simulink model "eqns_motion_mdl"  (R2018b)
settings: Solver=VariableStepAuto  StartTime=0.0  StopTime=200  FixedStep=0.001  RelTol=1e-4
values from neighbouring files (symbols this model uses):
  air_data = load('air_data.csv')    [Saturn_V_Comp2.m]    (also in eqns_motion_script.m)
  burn_time = 153.82    [Saturn_V_Comp2.m]    (also in eqns_motion_script.m = 39.2157)
  cp = 0.217    [Saturn_V_Comp2.m]    (also in draw_vehicle.m = -aero_statdyn.xcp(alpha, 1)*aero_statdyn.cbar + vehicle.xcg; eqns_motion_script.m)
  d = 16    [Saturn_V_Comp2.m]    (also in eqns_motion_script.m)
  De = 12.2*12    (= 146.4)    [Saturn_V_Comp2.m]    (also in eqns_motion_script.m = 8.4932)
  h0 = 10    [Saturn_V_Comp2.m]    (also in eqns_motion_script.m = 4595)
  I = [360, 0, 0; 0, 4880, 0; 0, 0, 4880]./973.065    [Saturn_V_Comp2.m]    (also in eqns_motion_script.m)
  k_he = 0.0867    [Saturn_V_Comp2.m]    (also in eqns_motion_script.m)
  kc = 1    [Saturn_V_Comp2.m]    (also in eqns_motion_script.m)
  lat = 32.9861    [Saturn_V_Comp2.m]    (also in eqns_motion_script.m)
  len = 27    [Saturn_V_Comp2.m]    (also in eqns_motion_script.m)
  lon = -106.9717    [Saturn_V_Comp2.m]    (also in eqns_motion_script.m)
  lr = 75    [Saturn_V_Comp2.m]    (also in eqns_motion_script.m)
  m_dry = 1.7664E6    (= 1766400)    [Saturn_V_Comp2.m]    (also in eqns_motion_script.m = 488.705562)
  m_wet = 6132585    [Saturn_V_Comp2.m]    (also in eqns_motion_script.m = 1404)
  material_density = 168.55    [Saturn_V_Comp2.m]    (also in eqns_motion_script.m)
  mu = 0.42    [Saturn_V_Comp2.m]    (also in eqns_motion_script.m)
  Pe = 13.3069    [Saturn_V_Comp2.m]    (also in eqns_motion_script.m = 10)
  phi0 = 0    [Saturn_V_Comp2.m]    (also in eqns_motion_script.m)
  psi0 = 0    [Saturn_V_Comp2.m]    (also in eqns_motion_script.m)
  tc = 0    [Saturn_V_Comp2.m]    (also in eqns_motion_script.m)
  theta0 = 0    [Saturn_V_Comp2.m]    (also in eqns_motion_script.m)
  u0 = 0.1    [Saturn_V_Comp2.m]    (also in eqns_motion_script.m)
  v0 = 0.0    (= 0)    [Saturn_V_Comp2.m]    (also in eqns_motion_script.m)
  w0 = 0    [Saturn_V_Comp2.m]    (also in eqns_motion_script.m)
  x = [0 10 15 20 40 60 80 100 120 140 150]    [Saturn_V_Comp2.m]    (also in draw_vehicle.m = linspace(0, vehicle.L_nc, 10)'; eqns_motion_script.m = 50.61)
undefined symbols (not defined in the file or in its folder): day, Dt, Earth, mdot, Pc, Receive, sec, Send, Thrust, WGS84
libraries: aerolibconvert2 x8, simulink_extras x5, vrlib x3, simulink x3, aerolibfltsims x2, aerolibasang x2, aerolibatmos2 x1, aerolibutil x1, aerolibtransform2 x1, aerolibadyn x1, sharedtransform x1, sharedutil x1
settings Model: Creator=Arthur de Waleffe  LastModifiedBy=bartk

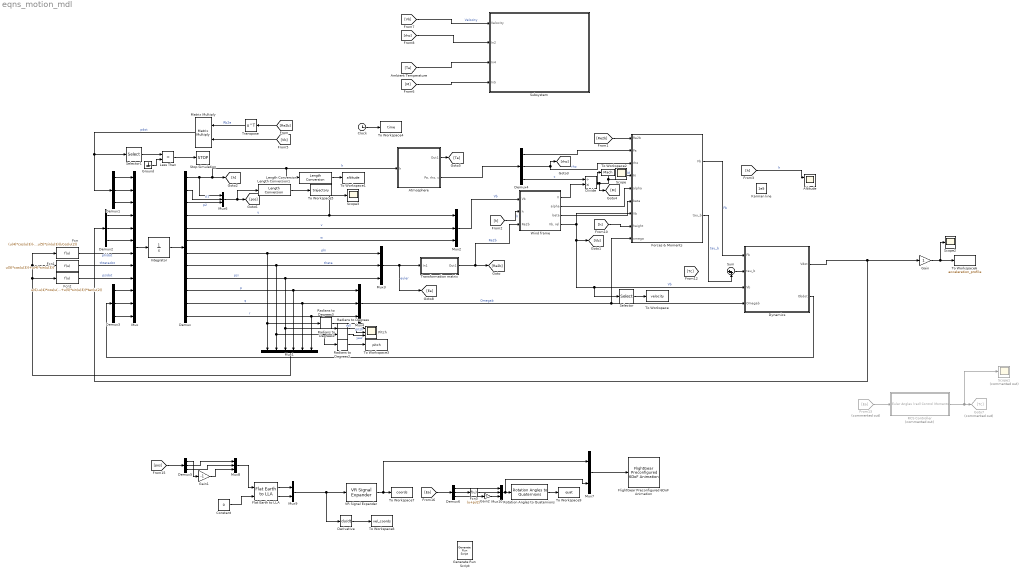
== system eqns_motion_mdl ==
  Altitude : Scope  NumInputPorts=2
  Atmosphere : Subsystem
  Clock : Clock
  Constant : Constant  Value=0
  Demux : Demux  Outputs=12
  Demux{1..6} (6 alike) : Demux  Outputs=3
  Derivative : Derivative
  Divide : Product  Inputs=/*
  Dynamics : Subsystem
  Fcn : Fcn  Expr=(u(4)*cos(u(3))-u(5)*sin(u(3)))/cos(u(2))
  Fcn1 : Fcn  Expr=u(5)*cos(u(3))+u(4)*sin(u(3))
  Fcn2 : Fcn  Expr=u(6)-u(4)*cos(u(3))*tan(u(2))+u(5)*sin(u(3))*tan(u(2))
  Fcn3 : Fcn  Expr=(u+pi/2)
  Flat Earth to LLA : aerolibtransform2/Flat Earth to LLA  units=Metric (MKS)  ptype=Earth (WGS84)  F=1/298.257223563  R=6378137  LL0=[lat lon]  psi=0
  FlightGear Preconfigured 6DoF Animation : aerolibfltsims/FlightGear Preconfigured 6DoF Animation  xFlightGearVersion=v2018.1  DestinationIpAddress=127.0.0.1  DestinationPort=5502  SampleTime=1/30  packetVersion=24
      settings: SourceProductName=Aerospace Blockset
  Forces & Moments : Subsystem
  From13 : From  Commented=on  GotoTag=Ea
  Gain : Gain
  Gain1 : Gain  Gain=-1
  Gain2 : Gain  Gain=-1
  Generate Run Script : aerolibfltsims/Generate Run Script  Architecture=Win64  dataFlow=Send-Receive  GeometryModelName=c172p  AirportId=KSFO  RunwayId=10L  InitialAltitude=h0  InitialHeading=0  OffsetDistance=0  OffsetAzimuth=0  InstallScenery=on  DisableShaders=off  OriginAddress=127.0.0.1  DestinationPort=5502  OriginPort=5505  LocalAddress=127.0.0.1  OutputFileName=runfg.bat  FlightGearBaseDirectory=C:\Program Files\FlightGear 2018.3.4
  Goto7 : Goto  Commented=on  GotoTag=Tc
  Ground : Ground
  Integrator : Integrator  InitialCondition=[h0*0.3048;0;0;u0*0.3048;v0*0.3048;w0*0.3048;phi0;theta0;psi0;0;0;0]
  Karman line : Constant  Value=1e5
  Length Conversion : aerolibconvert2/Length Conversion  IU=m  OU=ft
  Length Conversion1 : aerolibconvert2/Length Conversion  IU=m  OU=ft
  Less Than : RelationalOperator  Operator=<  OutDataTypeStr=boolean  RndMeth=Simplest
  Matrix Multiply : Product  Multiplication=Matrix(*)
  Mux : Mux  Inputs=12
  Mux1 : Mux  Inputs=6
  Mux{2..4,6,8,10} (6 alike) : Mux  Inputs=3
  Mux7 : Mux  Inputs=2
  Mux9 : Mux  Inputs=2
  Pitch : Scope  NumInputPorts=3
  RCS Controller : Subsystem  Commented=on
  Radians to Degrees{,1..3} (4 alike) : simulink_extras/Transformations/Radians to Degrees
  Rotation Angles to Quaternions : sharedtransform/Rotation Angles to Quaternions  rotationOrder=ZYX  aMode=aMode
      settings: SourceProductName=Aerospace Blockset  SourceProductBaseCode=AE
  Scope : Scope
  Scope1 : Scope  Commented=on
  Scope2 : Scope
  Scope3 : Scope
  Selector : Selector  InputPortWidth=3  IndexOptions=Index vector (dialog)  Indices=[1]  OutputSizes=1
  Selector1 : Selector  InputPortWidth=3  IndexOptions=Index vector (dialog)  Indices=[1]  OutputSizes=1
  Stop Simulation : Stop
  Subsystem : Subsystem
  Sum : Sum  Inputs=|++
  To Workspace : ToWorkspace  VariableName=velocity  SaveFormat=Timeseries  SampleTime=-1
  To Workspace1 : ToWorkspace  VariableName=altitude  SaveFormat=Timeseries  SampleTime=-1
  To Workspace2 : ToWorkspace  VariableName=Mach  SaveFormat=Timeseries  SampleTime=-1
  To Workspace3 : ToWorkspace  VariableName=pitch  SaveFormat=Timeseries  SampleTime=-1
  To Workspace4 : ToWorkspace  VariableName=time  SampleTime=-1
  To Workspace5 : ToWorkspace  VariableName=trajectory  SaveFormat=Timeseries  SampleTime=-1
  To Workspace6 : ToWorkspace  VariableName=acceleration_profile  SampleTime=-1
  To Workspace7 : ToWorkspace  VariableName=coords  SaveFormat=Structure With Time  SampleTime=-1
  To Workspace8 : ToWorkspace  VariableName=vel_coords  SaveFormat=Structure With Time  SampleTime=-1
  To Workspace9 : ToWorkspace  VariableName=quat  SaveFormat=Structure With Time  SampleTime=-1
  Transformation matrix : Subsystem
  Transpose : Math  Operator=transpose  SaturateOnIntegerOverflow=on
  VR Signal Expander : vrlib/VR Signal Expander  outwidth=3  outidx=[2 1 3]
      settings: SourceProductName=Simulink 3D Animation  SourceProductBaseCode=VR
  "Wind frame " : Subsystem
  wires:
  Integrator/1 -> Demux/1
  Mux/1 -> Integrator/1
  Demux/4 -> Scope3/1, Mux2/1  "u"
  Demux/5 -> Mux2/2  "v"
  Demux/6 -> Mux2/3  "w"
  Demux/7 -> Mux3/1, Mux1/1, Radians to Degrees3/1  "phi"
  Demux/8 -> Mux3/2, Radians to Degrees2/1, Radians to Degrees1/1, Mux1/2  "theta"
  Demux/9 -> Mux3/3, Mux1/3, Radians to Degrees/1  "psi"
  Demux/10 -> Mux4/1, Mux1/4  "p"
  Demux/12 -> Mux4/3, Mux1/6  "r"
  Demux/11 -> Mux4/2, Mux1/5  "q"
  Fcn/1 -> Mux/7  "phidot"
  Fcn1/1 -> Mux/8  "thtetadot"
  Fcn2/1 -> Mux/9  "psidot"
  Mux1/1 -> Fcn2/1, Fcn/1, Fcn1/1
  Mux3/1 -> [Ea], Transformation matrix/1(In1)  "euler"
  Transpose/1 -> Matrix Multiply/1  "Rb2e"
  Matrix Multiply/1 -> Selector1/1, Demux1/1  "pdot"
  Demux1/2 -> Mux/2
  Demux1/1 -> Mux/1
  Demux1/3 -> Mux/3
  Demux2/1 -> Mux/4
  Demux2/2 -> Mux/5
  Demux2/3 -> Mux/6
  Demux4/2 -> [rho], Forces & Moments/3(rho)  "rho"
  Demux3/1 -> Mux/10
  Demux3/2 -> Mux/11
  Demux3/3 -> Mux/12
  Demux4/3 -> Divide/1  "c"
  Divide/1 -> To Workspace2/1, [M], Scope/1, Forces & Moments/4(M)  "M"
  "Wind frame "/1(V) -> Divide/2
  "Wind frame "/2(alpha) -> Forces & Moments/5(alpha)
  "Wind frame "/3(beta) -> Forces & Moments/6(beta)
  Demux/2 -> Mux6/2  "p1"
  Demux/3 -> Mux6/3  "p2"
  Forces & Moments/1(Fb) -> Dynamics/1(Fb)  "Fb"
  Mux4/1 -> Forces & Moments/9(omega), Dynamics/4(Omegab)  "Omegab"
  Transformation matrix/1(Out1) -> "Wind frame "/3(Re2b), [Re2b]  "Re2b"
  [Re2b] -> Transpose/1
  [Re2b] -> Forces & Moments/1(Re2b)
  [Vb] -> Matrix Multiply/2
  [h] -> Altitude/1  "h"
  "Wind frame "/4("Vb, rel") -> [Vb], Selector/1, Dynamics/3(Vb), Forces & Moments/7(Vb)  "Vb"
  Mux2/1 -> "Wind frame "/1(Vb)  "Vb"
  Demux4/1 -> Forces & Moments/2(Pa)
  Atmosphere/2("Pa, rho, c") -> Demux4/1
  Demux/1 -> Mux6/1, Length Conversion/1, Atmosphere/1(h), [h]  "h"
  [h] -> "Wind frame "/2(h)  "h"
  [Ta] -> Subsystem/3(In4)
  [Vb] -> Subsystem/1(Velocity)  "Velocity"
  [M] -> Subsystem/4(In5)
  [rho] -> Subsystem/2(In2)
  Atmosphere/1(Out1) -> [Ta]
  [h] -> Forces & Moments/8(height)
  Mux6/1 -> Length Conversion1/1, [pos]
  Radians to Degrees/1 -> Pitch/2  "pitch"
  Radians to Degrees1/1 -> Pitch/3  "yaw"
  Radians to Degrees2/1 -> To Workspace3/1
  Clock/1 -> To Workspace4/1
  From13/1 -> RCS Controller/1(Euler Angles (rad))
  Dynamics/2(Obdot) -> Demux3/1
  RCS Controller/1(Control Moments) -> Scope1/1, Goto7/1
  Sum/1 -> Dynamics/2(tau_b)
  Selector/1 -> To Workspace/1
  Dynamics/1(Vdot) -> Demux2/1, Gain/1
  Gain/1 -> Scope2/1, To Workspace6/1
  Constant/1 -> Flat Earth to LLA/2
  [pos] -> Demux5/1
  Demux5/2 -> Mux8/1
  Demux5/3 -> Mux8/2
  Demux5/1 -> Gain1/1
  Gain1/1 -> Mux8/3
  Mux8/1 -> Flat Earth to LLA/1
  Flat Earth to LLA/1 -> Mux9/1
  Flat Earth to LLA/2 -> Mux9/2
  Mux9/1 -> Derivative/1, VR Signal Expander/1
  Derivative/1 -> To Workspace8/1
  [Ea] -> Demux6/1
  Demux6/1 -> Mux10/1
  Mux10/1 -> Mux7/2, Rotation Angles to Quaternions/1
  Demux6/2 -> Fcn3/1
  Demux6/3 -> Gain2/1
  Fcn3/1 -> Mux10/2
  Gain2/1 -> Mux10/3
  Ground/1 -> Less Than/2
  Less Than/1 -> Stop Simulation/1
  Rotation Angles to Quaternions/1 -> To Workspace9/1
  Radians to Degrees3/1 -> Pitch/1  "roll"
  VR Signal Expander/1 -> Mux7/1, To Workspace7/1
  Mux7/1 -> FlightGear Preconfigured 6DoF Animation/1
  Forces & Moments/2(tau_b) -> Sum/2  "tau_b"
  Length Conversion/1 -> To Workspace1/1
  Length Conversion1/1 -> To Workspace5/1
  Selector1/1 -> Less Than/1

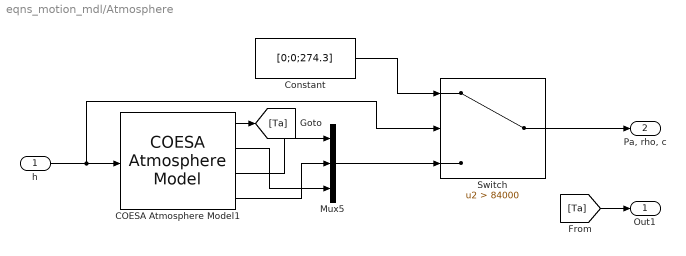
== system eqns_motion_mdl/Atmosphere ==
  h : Inport
  COESA Atmosphere Model1 : aerolibatmos2/COESA Atmosphere Model  units=Metric (MKS)  spec=1976 COESA-extended U.S. Standard Atmosphere  model=Profile  profile_var=High temperature  profile_percent=1%  profile_alt=5 km (16404 ft)  envelope_var=High temperature  envelope_percent=1%  action=Warning
  Constant : Constant  Value=[0;0;274.3]
  Mux5 : Mux  Inputs=3
  Switch : Switch  Criteria=u2 > Threshold  Threshold=84000
  Out1 : Outport
  "Pa, rho, c" : Outport  Port=2
  wires:
  Switch/1 -> "Pa, rho, c"/1
  COESA Atmosphere Model1/3 -> Mux5/1
  Constant/1 -> Switch/1
  Mux5/1 -> Switch/3
  COESA Atmosphere Model1/1 -> [Ta]
  COESA Atmosphere Model1/4 -> Mux5/2
  COESA Atmosphere Model1/2 -> Mux5/3
  h/1 -> COESA Atmosphere Model1/1, Switch/2
  [Ta] -> Out1/1

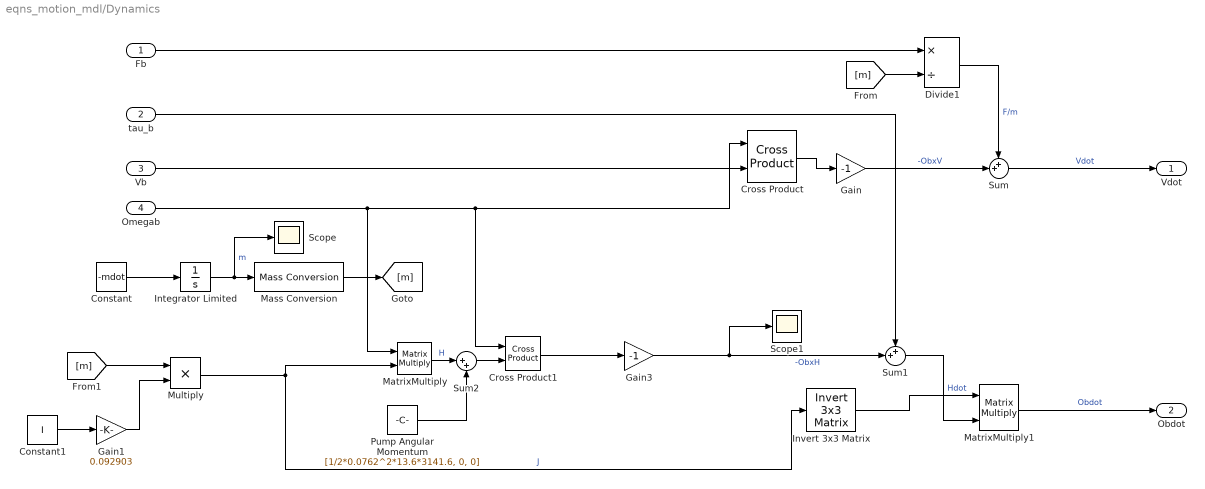
== system eqns_motion_mdl/Dynamics ==
  Fb : Inport
  tau_b : Inport  Port=2
  Vb : Inport  Port=3
  Omegab : Inport  Port=4
  Constant : Constant  Value=-mdot
  Constant1 : Constant  Value=I
  Cross Product : vrlib/Utilities/Cross Product
      settings: SourceProductBaseCode=VR
  Cross Product1 : vrlib/Utilities/Cross Product
      settings: SourceProductBaseCode=VR
  Divide1 : Product  Inputs=*/
  Gain : Gain  Gain=-1
  Gain1 : Gain  Gain=0.092903
  Gain3 : Gain  Gain=-1
  Integrator Limited : Integrator  InitialCondition=m_wet  LimitOutput=on  UpperSaturationLimit=m_wet  LowerSaturationLimit=m_dry
  Invert 3x3 Matrix : aerolibutil/Invert  3x3 Matrix
  Mass Conversion : aerolibconvert2/Mass Conversion  IU=lbm  OU=kg
      settings: SourceProductName=Aerospace Blockset  SourceProductBaseCode=AE
  MatrixMultiply : Product  Multiplication=Matrix(*)
  MatrixMultiply1 : Product  Multiplication=Matrix(*)
  Multiply : Product
  Pump Angular Momentum : Constant  Value=[1/2*0.0762^2*13.6*3141.6, 0, 0]
  Scope : Scope
  Scope1 : Scope
  Sum : Sum  Inputs=++|
  Sum1 : Sum  Inputs=++|
  Sum2 : Sum  Inputs=|++
  Vdot : Outport
  Obdot : Outport  Port=2
  wires:
  Multiply/1 -> MatrixMultiply/2, Invert 3x3 Matrix/1  "J"
  MatrixMultiply1/1 -> Obdot/1  "Obdot"
  Cross Product/1 -> Gain/1
  Sum1/1 -> MatrixMultiply1/2  "Hdot"
  Integrator Limited/1 -> Scope/1, Mass Conversion/1  "m"
  Gain3/1 -> Scope1/1, Sum1/2  "-ObxH"
  Cross Product1/1 -> Gain3/1
  Omegab/1 -> Cross Product/1, Cross Product1/1, MatrixMultiply/1
  Gain/1 -> Sum/2  "-ObxV"
  Invert 3x3 Matrix/1 -> MatrixMultiply1/1
  Sum/1 -> Vdot/1  "Vdot"
  Divide1/1 -> Sum/1  "F/m"
  Vb/1 -> Cross Product/2
  Fb/1 -> Divide1/1
  tau_b/1 -> Sum1/1
  [m] -> Divide1/2
  [m] -> Multiply/1
  Constant/1 -> Integrator Limited/1
  MatrixMultiply/1 -> Sum2/1  "H"
  Sum2/1 -> Cross Product1/2
  Pump Angular Momentum/1 -> Sum2/2
  Mass Conversion/1 -> [m]
  Constant1/1 -> Gain1/1
  Gain1/1 -> Multiply/2

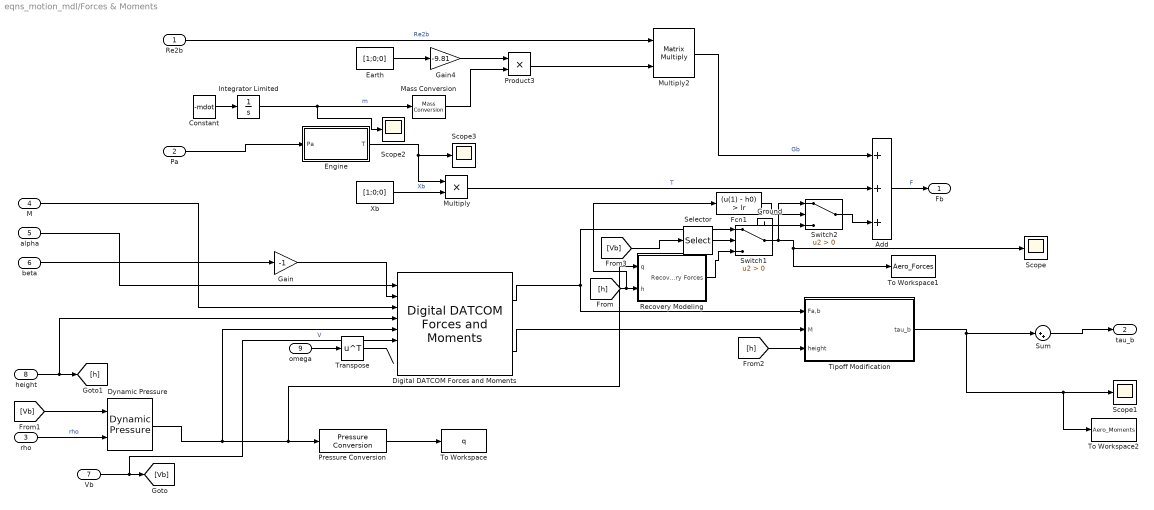
== system eqns_motion_mdl/Forces & Moments ==
  Re2b : Inport
  Pa : Inport  Port=2
  rho : Inport  Port=3
  M : Inport  Port=4
  alpha : Inport  Port=5
  beta : Inport  Port=6
  Vb : Inport  Port=7
  height : Inport  Port=8
  omega : Inport  Port=9
  Add : Sum  Inputs=+++
  Constant : Constant  Value=-mdot
  Digital DATCOM Forces and Moments : aerolibadyn/Digital DATCOM Forces and Moments  units=Metric (MKS)  dcase=aero_statdyn  fmode=Body  buildno=0  imethod=Linear  emethod=Linear  rmethod=Linear Extrapolation  action=None
      settings: SourceProductName=Aerospace Blockset  SourceProductBaseCode=AE
  Dynamic Pressure : aerolibasang/Dynamic Pressure
  Earth : Constant  Value=[1;0;0]
  Engine : Subsystem
  Fcn1 : Fcn  Expr=(u(1) - h0) > lr
  Gain : Gain  Gain=-1
  Gain4 : Gain  Gain=-9.81
  Ground : Ground
  Integrator Limited : Integrator  InitialCondition=m_wet  LimitOutput=on  UpperSaturationLimit=m_wet  LowerSaturationLimit=m_dry
  Mass Conversion : aerolibconvert2/Mass Conversion  IU=lbm  OU=kg
      settings: SourceProductName=Aerospace Blockset  SourceProductBaseCode=AE
  Multiply : Product
  Multiply2 : Product  Multiplication=Matrix(*)
  Pressure Conversion : aerolibconvert2/Pressure Conversion  IU=Pa  OU=psf
      settings: SourceProductName=Aerospace Blockset  SourceProductBaseCode=AE
  Product3 : Product
  Recovery Modeling : Subsystem
  Scope{,1..3} (4 alike) : Scope
  Selector : Selector  InputPortWidth=3  IndexOptions=Index vector (dialog)  Indices=[1]  OutputSizes=1
  Sum : Sum  Inputs=|++
  Switch1 : Switch  Criteria=u2 > Threshold
  Switch2 : Switch  Criteria=u2 > Threshold
  Tipoff Modification : Subsystem
  To Workspace : ToWorkspace  VariableName=q  SaveFormat=Timeseries  SampleTime=-1
  To Workspace1 : ToWorkspace  VariableName=Aero_Forces  SaveFormat=Timeseries  SampleTime=-1
  To Workspace2 : ToWorkspace  VariableName=Aero_Moments  SaveFormat=Timeseries  SampleTime=-1
  Transpose : Math  Operator=transpose  SaturateOnIntegerOverflow=on
  Xb : Constant  Value=[1;0;0]
  Fb : Outport
  tau_b : Outport  Port=2
  wires:
  Multiply2/1 -> Add/1  "Gb"
  Re2b/1 -> Multiply2/1  "Re2b"
  Earth/1 -> Gain4/1
  Add/1 -> Fb/1  "F"
  Gain4/1 -> Product3/1
  Integrator Limited/1 -> Mass Conversion/1, Scope2/1  "m"
  Product3/1 -> Multiply2/2
  Xb/1 -> Multiply/2  "Xb"
  Multiply/1 -> Add/2  "T"
  rho/1 -> Dynamic Pressure/2  "rho"
  [Vb] -> Dynamic Pressure/1
  Pa/1 -> Engine/1(Pa)
  Engine/1(T) -> Scope3/1, Multiply/1
  [h] -> Tipoff Modification/3(height)
  height/1 -> Digital DATCOM Forces and Moments/4, [h]
  Vb/1 -> Digital DATCOM Forces and Moments/6, [Vb]  "V"
  Dynamic Pressure/1 -> Digital DATCOM Forces and Moments/5, Recovery Modeling/1(q), Pressure Conversion/1
  M/1 -> Digital DATCOM Forces and Moments/3
  alpha/1 -> Digital DATCOM Forces and Moments/1
  beta/1 -> Gain/1
  Gain/1 -> Digital DATCOM Forces and Moments/2
  omega/1 -> Transpose/1
  Digital DATCOM Forces and Moments/2 -> Tipoff Modification/2(M)
  Digital DATCOM Forces and Moments/1 -> Switch1/1, Tipoff Modification/1(Fa,b)
  Transpose/1 -> ?
  Tipoff Modification/1(tau_b) -> Sum/1, Scope1/1, To Workspace2/1
  Switch1/1 -> Switch2/1, To Workspace1/1, Scope/1
  Recovery Modeling/1(Recovery Forces) -> Switch1/3
  [h] -> Fcn1/1, Recovery Modeling/2(h)
  [Vb] -> Selector/1
  Selector/1 -> Switch1/2
  Pressure Conversion/1 -> To Workspace/1
  Fcn1/1 -> Switch2/2
  Ground/1 -> Switch2/3
  Constant/1 -> Integrator Limited/1
  Mass Conversion/1 -> Product3/2
  Switch2/1 -> Add/3
  Sum/1 -> tau_b/1

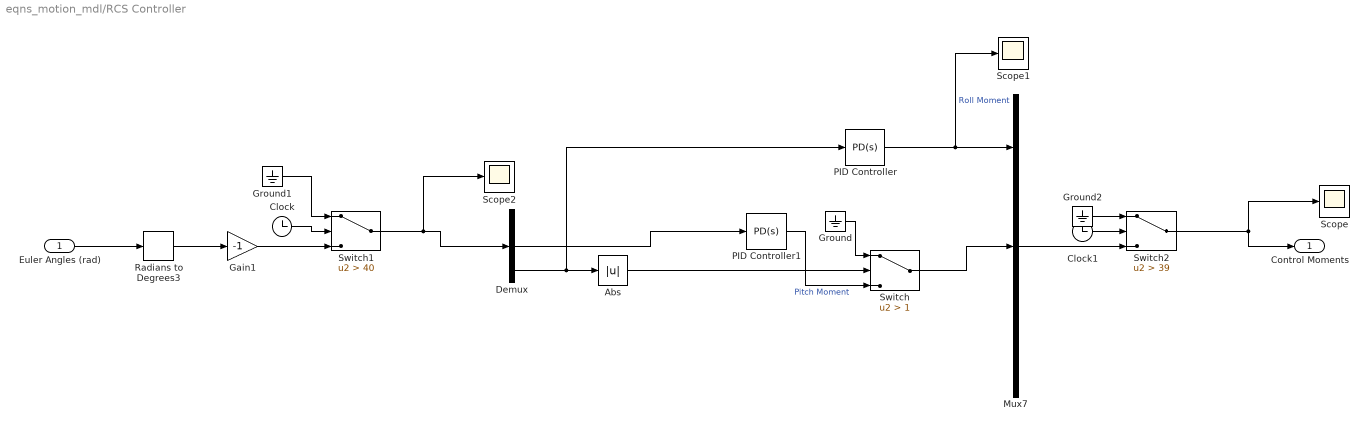
== system eqns_motion_mdl/RCS Controller ==
  Euler Angles (rad) : Inport
  Abs : Abs
  Clock : Clock
  Clock1 : Clock
  Demux : Demux  Outputs=3
  Gain1 : Gain  Gain=-1
  Ground : Ground
  Ground1 : Ground
  Ground2 : Ground
  Mux7 : Mux  Inputs=3
  PID Controller : simulink/Continuous/PID Controller  Controller=PD  Form=Parallel  TimeDomain=Continuous-time  SampleTime=-1  IntegratorMethod=Forward Euler  FilterMethod=Forward Euler  ControllerParametersSource=internal  P=2  I=1  D=2  UseFilter=on  N=100  TunerSelectOption=Transfer Function Based (PID Tuner App)  InitialConditionSource=internal  InitialConditionForIntegrator=0  InitialConditionForFilter=0  DifferentiatorICPrevScaledInput=0  ExternalReset=none  TrackingMode=off  Kt=1  LimitOutput=off  UpperSaturationLimit=inf  LowerSaturationLimit=-inf  LinearizeAsGain=on  AntiWindupMode=none  Kb=1  POutMin=[]  POutMax=[]  IOutMin=[]  IOutMax=[]  DOutMin=[]  DOutMax=[]  NOutMin=[]  NOutMax=[]  SumOutMin=[]  SumOutMax=[]  SaturationOutMin=[]  SaturationOutMax=[]  PParamMin=[]  PParamMax=[]  IParamMin=[]  IParamMax=[]  DParamMin=[]  DParamMax=[]  NParamMin=[]  NParamMax=[]  KbParamMin=[]  KbParamMax=[]  KtParamMin=[]  KtParamMax=[]  KbOutMin=[]  KbOutMax=[]  KtOutMin=[]  KtOutMax=[]  IntegratorOutMin=[]  IntegratorOutMax=[]  FilterOutMin=[]  FilterOutMax=[]  SumI1OutMin=[]  SumI1OutMax=[]  SumI2OutMin=[]  SumI2OutMax=[]  SumI3OutMin=[]  SumI3OutMax=[]  SumI4OutMin=[]  SumI4OutMax=[]  SumDOutMin=[]  SumDOutMax=[]  DifferentiatorOutMin=[]  DifferentiatorOutMax=[]  FilterDiffOutCoefMin=[]  FilterDiffOutCoefMax=[]  ReciprocalOutMin=[]  ReciprocalOutMax=[]  SumDenOutMin=[]  SumDenOutMax=[]  SumNumOutMin=[]  SumNumOutMax=[]  DivideOutMin=[]  DivideOutMax=[]  IntegratorContinuousStateAttributes=''  IntegratorStateMustResolveToSignalObject=off  IntegratorRTWStateStorageClass=Auto  FilterContinuousStateAttributes=''  FilterStateMustResolveToSignalObject=off  FilterRTWStateStorageClass=Auto  ParallelPVariant=InternalParameters  IdealPVariant=Disabled  IVariant=Disabled  DVariant=InternalParameters  IntegratorVariant=Disabled  SatVariant=Disabled  AWVariant=Disabled  PCopyVariant=Disabled  TRVariant=Disabled  FdbkBlocksVariant=Forward  IdealPFdbkVariant=Disabled  SatFdbkVariant=Disabled  DerivativeFilterVariant=ContFilter  NVariant=InternalParameters  NCopyVariant=Disabled  FilterICVariant=InternalICsFilter  IntegratorICVariant=Disabled  ExternalResetVariant=Disabled  TRSumVariant=Passthrough  SumFdbkVariant=Disabled  SumVariant=Sum_PD
  PID Controller1 : simulink/Continuous/PID Controller  Controller=PD  Form=Parallel  TimeDomain=Continuous-time  SampleTime=-1  IntegratorMethod=Forward Euler  FilterMethod=Forward Euler  ControllerParametersSource=internal  P=1281.40350850482  I=1  D=624.70270979077  UseFilter=on  N=100  TunerSelectOption=Transfer Function Based (PID Tuner App)  InitialConditionSource=internal  InitialConditionForIntegrator=0  InitialConditionForFilter=0  DifferentiatorICPrevScaledInput=0  ExternalReset=none  TrackingMode=off  Kt=1  LimitOutput=on  UpperSaturationLimit=1000  LowerSaturationLimit=-1000  LinearizeAsGain=on  AntiWindupMode=none  Kb=1  POutMin=[]  POutMax=[]  IOutMin=[]  IOutMax=[]  DOutMin=[]  DOutMax=[]  NOutMin=[]  NOutMax=[]  SumOutMin=[]  SumOutMax=[]  SaturationOutMin=[]  SaturationOutMax=[]  PParamMin=[]  PParamMax=[]  IParamMin=[]  IParamMax=[]  DParamMin=[]  DParamMax=[]  NParamMin=[]  NParamMax=[]  KbParamMin=[]  KbParamMax=[]  KtParamMin=[]  KtParamMax=[]  KbOutMin=[]  KbOutMax=[]  KtOutMin=[]  KtOutMax=[]  IntegratorOutMin=[]  IntegratorOutMax=[]  FilterOutMin=[]  FilterOutMax=[]  SumI1OutMin=[]  SumI1OutMax=[]  SumI2OutMin=[]  SumI2OutMax=[]  SumI3OutMin=[]  SumI3OutMax=[]  SumI4OutMin=[]  SumI4OutMax=[]  SumDOutMin=[]  SumDOutMax=[]  DifferentiatorOutMin=[]  DifferentiatorOutMax=[]  FilterDiffOutCoefMin=[]  FilterDiffOutCoefMax=[]  ReciprocalOutMin=[]  ReciprocalOutMax=[]  SumDenOutMin=[]  SumDenOutMax=[]  SumNumOutMin=[]  SumNumOutMax=[]  DivideOutMin=[]  DivideOutMax=[]  IntegratorContinuousStateAttributes=''  IntegratorStateMustResolveToSignalObject=off  IntegratorRTWStateStorageClass=Auto  FilterContinuousStateAttributes=''  FilterStateMustResolveToSignalObject=off  FilterRTWStateStorageClass=Auto  ParallelPVariant=InternalParameters  IdealPVariant=Disabled  IVariant=Disabled  DVariant=InternalParameters  IntegratorVariant=Disabled  SatVariant=Enabled  AWVariant=Disabled  PCopyVariant=Disabled  TRVariant=Disabled  FdbkBlocksVariant=Forward  IdealPFdbkVariant=Disabled  SatFdbkVariant=Disabled  DerivativeFilterVariant=ContFilter  NVariant=InternalParameters  NCopyVariant=Disabled  FilterICVariant=InternalICsFilter  IntegratorICVariant=Disabled  ExternalResetVariant=Disabled  TRSumVariant=Passthrough  SumFdbkVariant=Disabled  SumVariant=Sum_PD
  Radians to Degrees3 : simulink_extras/Transformations/Radians to Degrees
  Scope : Scope
  Scope1 : Scope
  Scope2 : Scope
  Switch : Switch  Criteria=u2 > Threshold  Threshold=1
  Switch1 : Switch  Criteria=u2 > Threshold  Threshold=40
  Switch2 : Switch  Criteria=u2 > Threshold  Threshold=39
  Control Moments : Outport
  wires:
  Radians to Degrees3/1 -> Gain1/1
  PID Controller/1 -> Scope1/1, Mux7/1  "Roll Moment"
  Euler Angles (rad)/1 -> Radians to Degrees3/1
  Demux/2 -> PID Controller1/1
  PID Controller1/1 -> Switch/3  "Pitch Moment"
  Ground/1 -> Switch/1
  Demux/3 -> PID Controller/1, Abs/1
  Abs/1 -> Switch/2
  Switch/1 -> Mux7/2
  Gain1/1 -> Switch1/3
  Switch1/1 -> Scope2/1, Demux/1
  Clock/1 -> Switch1/2
  Ground1/1 -> Switch1/1
  Mux7/1 -> Switch2/3
  Switch2/1 -> Control Moments/1, Scope/1
  Clock1/1 -> Switch2/2
  Ground2/1 -> Switch2/1

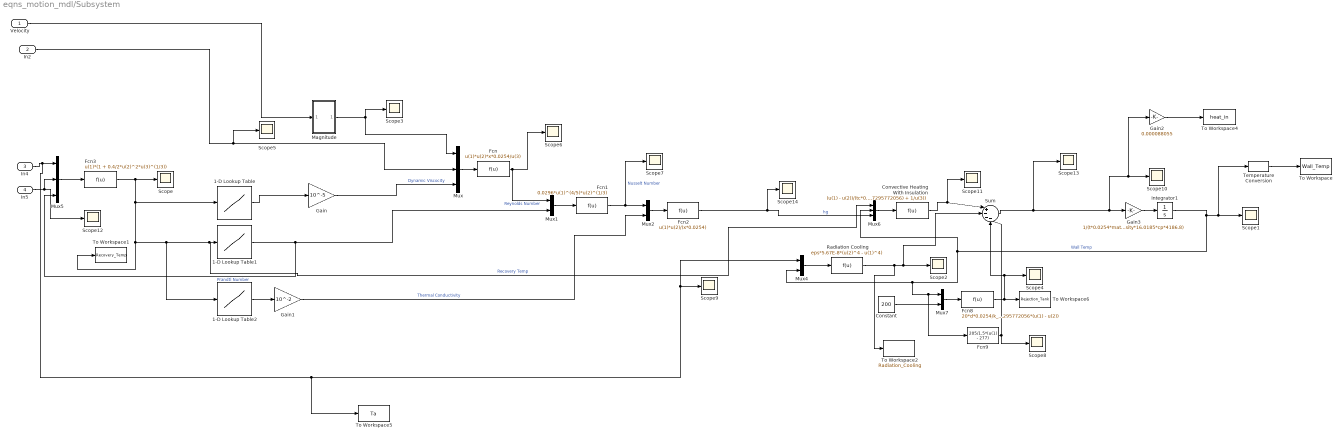
== system eqns_motion_mdl/Subsystem ==
  Velocity : Inport
  In2 : Inport  Port=2
  In4 : Inport  Port=3
  In5 : Inport  Port=4
  1-D Lookup Table : Lookup_n-D  NumberOfTableDimensions=1  BreakpointsForDimension1=air_data(:,1)  Table=air_data(:,5)  InternalRulePriority=Speed  RndMeth=Simplest  InputSameDT=on
  1-D Lookup Table1 : Lookup_n-D  NumberOfTableDimensions=1  BreakpointsForDimension1=air_data(:,1)  Table=air_data(:,7)  InternalRulePriority=Speed  RndMeth=Simplest  InputSameDT=on
  1-D Lookup Table2 : Lookup_n-D  NumberOfTableDimensions=1  BreakpointsForDimension1=air_data(:,1)  Table=air_data(:,6)  InternalRulePriority=Speed  RndMeth=Simplest  InputSameDT=on
  Constant : Constant  Value=200
  Convective Heating With Insulation : Fcn  Expr=(u(1) - u(2))/(tc*0.0254/(kc*1.7295772056) + 1/u(3))
  Fcn : Fcn  Expr=u(1)*u(2)*x*0.0254/u(3)
  Fcn1 : Fcn  Expr=0.0296*u(1)^(4/5)*u(2)^(1/3)
  Fcn2 : Fcn  Expr=u(1)*u(2)/(x*0.0254)
  Fcn3 : Fcn  Expr=u(1)*(1 + 0.4/2*u(2)^2*u(3)^(1/3))
  Fcn8 : Fcn  Expr=20*d*0.0254/k_he/1.7295772056*(u(1) - u(2))
  Fcn9 : Fcn  Expr=205/1.5*(u(1) - 277)
  Gain : Gain  Gain=10^-5
  Gain1 : Gain  Gain=10^-2
  Gain2 : Gain  Gain=0.000088055
  Gain3 : Gain  Gain=1/(t*0.0254*material_density*16.0185*cp*4186.8)
  Integrator1 : Integrator  InitialCondition=277
  Magnitude : Subsystem
  Mux : Mux  Inputs=3
  Mux{1..2,4,7} (4 alike) : Mux  Inputs=2
  Mux5 : Mux  Inputs=3
  Mux6 : Mux  Inputs=3
  Radiation Cooling : Fcn  Expr=eps*5.67E-8*(u(2)^4 - u(1)^4)
  Scope{,1..14} (15 alike) : Scope
  Sum : Sum  Inputs=|+---
  Temperature Conversion : aerolibconvert2/Temperature Conversion  IU=K  OU=F
      settings: SourceProductName=Aerospace Blockset  SourceProductBaseCode=AE
  To Workspace : ToWorkspace  VariableName=Wall_Temp  SaveFormat=Timeseries  SampleTime=-1
  To Workspace1 : ToWorkspace  VariableName=Recovery_Temp  SaveFormat=Timeseries  SampleTime=-1
  To Workspace2 : ToWorkspace  VariableName=Radiation_Cooling  SaveFormat=Timeseries  SampleTime=-1
  To Workspace4 : ToWorkspace  VariableName=heat_in  SaveFormat=Structure With Time  SampleTime=-1
  To Workspace5 : ToWorkspace  VariableName=Ta  SaveFormat=Timeseries  SampleTime=-1
  To Workspace6 : ToWorkspace  VariableName=Rejection_Tank  SaveFormat=Timeseries  SampleTime=-1
  wires:
  Gain1/1 -> Mux2/2  "Thermal Conductivity"
  Mux5/1 -> Fcn3/1
  Fcn3/1 -> To Workspace1/1, 1-D Lookup Table2/1, Mux6/1, 1-D Lookup Table1/1, 1-D Lookup Table/1, Scope/1  "Recovery Temp"
  1-D Lookup Table1/1 -> Mux1/2, Mux5/3  "Prandtl Number"
  In2/1 -> Mux/2, Scope5/1
  1-D Lookup Table2/1 -> Gain1/1
  Gain/1 -> Mux/3  "Dynamic Viscocity"
  Integrator1/1 -> Mux6/2, Fcn9/1, Mux7/1, Mux4/2, Temperature Conversion/1, Scope1/1  "Wall Temp"
  In5/1 -> Scope12/1, Mux5/2
  Magnitude/1(Out1) -> Mux/1, Scope3/1
  1-D Lookup Table/1 -> Gain/1
  Velocity/1 -> Magnitude/1(Velocity)
  In4/1 -> To Workspace5/1, Scope9/1, Mux4/1, Mux5/1
  Mux/1 -> Fcn/1
  Fcn/1 -> Mux1/1, Scope6/1  "Reynolds Number"
  Mux1/1 -> Fcn1/1
  Fcn1/1 -> Scope7/1, Mux2/1  "Nusselt Number"
  Mux2/1 -> Fcn2/1
  Radiation Cooling/1 -> To Workspace2/1, Sum/2, Scope2/1
  Mux4/1 -> Radiation Cooling/1
  Gain3/1 -> Integrator1/1
  Convective Heating With Insulation/1 -> Scope11/1, Sum/1
  Mux6/1 -> Convective Heating With Insulation/1
  Mux7/1 -> Fcn8/1
  Fcn8/1 -> To Workspace6/1, Scope4/1, Sum/4
  Sum/1 -> Scope13/1, Gain2/1, Scope10/1, Gain3/1
  Temperature Conversion/1 -> To Workspace/1
  Gain2/1 -> To Workspace4/1
  Fcn9/1 -> Scope8/1, Sum/3
  Fcn2/1 -> Scope14/1, Mux6/3  "hg"
  Constant/1 -> Mux7/2

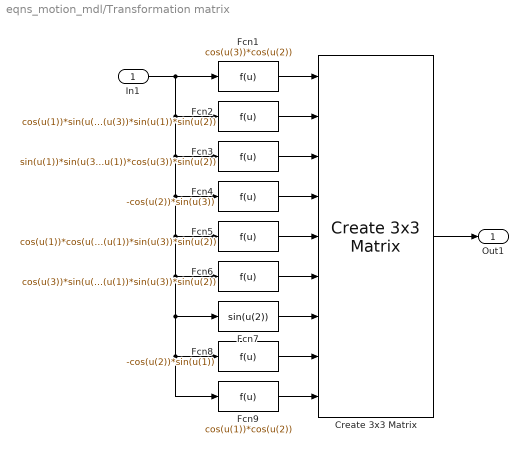
== system eqns_motion_mdl/Transformation matrix ==
  In1 : Inport
  Create 3x3 Matrix : sharedutil/Create 3x3 Matrix  aMode=aMode
  Fcn1 : Fcn  Expr=cos(u(3))*cos(u(2))
  Fcn2 : Fcn  Expr=cos(u(1))*sin(u(3)) + cos(u(3))*sin(u(1))*sin(u(2))
  Fcn3 : Fcn  Expr=sin(u(1))*sin(u(3)) - cos(u(1))*cos(u(3))*sin(u(2))
  Fcn4 : Fcn  Expr=-cos(u(2))*sin(u(3))
  Fcn5 : Fcn  Expr=cos(u(1))*cos(u(3)) - sin(u(1))*sin(u(3))*sin(u(2))
  Fcn6 : Fcn  Expr=cos(u(3))*sin(u(1)) + cos(u(1))*sin(u(3))*sin(u(2))
  Fcn7 : Fcn  Expr=sin(u(2))
  Fcn8 : Fcn  Expr=-cos(u(2))*sin(u(1))
  Fcn9 : Fcn  Expr=cos(u(1))*cos(u(2))
  Out1 : Outport
  wires:
  In1/1 -> Fcn9/1, Fcn8/1, Fcn7/1, Fcn6/1, Fcn5/1, Fcn4/1, Fcn3/1, Fcn2/1, Fcn1/1
  Fcn9/1 -> Create 3x3 Matrix/9
  Fcn8/1 -> Create 3x3 Matrix/8
  Fcn7/1 -> Create 3x3 Matrix/7
  Fcn6/1 -> Create 3x3 Matrix/6
  Fcn5/1 -> Create 3x3 Matrix/5
  Fcn4/1 -> Create 3x3 Matrix/4
  Fcn3/1 -> Create 3x3 Matrix/3
  Fcn2/1 -> Create 3x3 Matrix/2
  Fcn1/1 -> Create 3x3 Matrix/1
  Create 3x3 Matrix/1 -> Out1/1

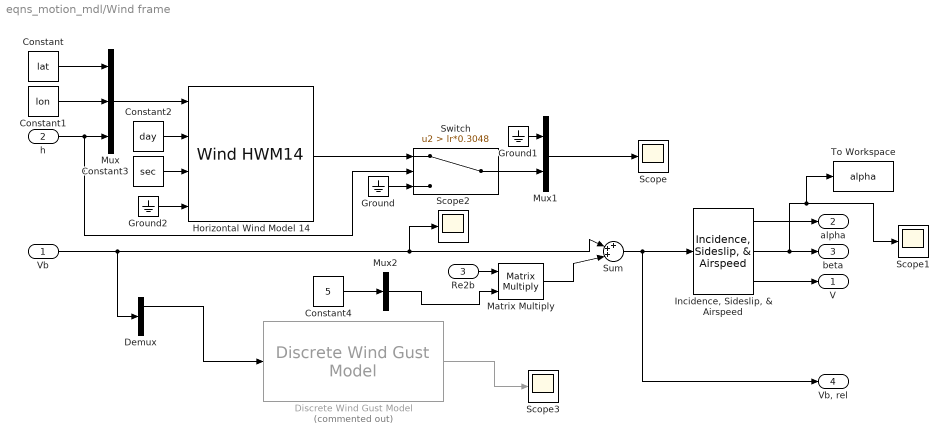
== system eqns_motion_mdl/Wind frame  ==
  Vb : Inport
  h : Inport  Port=2
  Re2b : Inport  Port=3
  Constant : Constant  Value=lat
  Constant1 : Constant  Value=lon
  Constant2 : Constant  Value=day
  Constant3 : Constant  Value=sec
  Constant4 : Constant  Value=5
  Demux : Demux  Outputs=3
  Discrete Wind Gust Model : aerolibwind2/Discrete Wind Gust Model  Commented=on  units=Metric (MKS)  Gx=off  Gy=on  Gz=off  t_0=17  d_m=[0 10 0]  v_m=[0 10 0]
      settings: SourceProductName=Aerospace Blockset
  Ground : Ground
  Ground1 : Ground
  Ground2 : Ground
  Horizontal Wind Model 14 : WindHWM14  model=Total  action=None
  "Incidence, Sideslip, & Airspeed" : aerolibasang/Incidence, Sideslip, & Airspeed
      settings: SourceProductName=Aerospace Blockset
  Matrix Multiply : Product  Multiplication=Matrix(*)
  Mux : Mux  Inputs=3
  Mux1 : Mux  Inputs=2
  Mux2 : Mux  Inputs=3
  Scope{,1..3} (4 alike) : Scope
  Sum : Sum  Inputs=+++|
  Switch : Switch  Criteria=u2 > Threshold  Threshold=lr*0.3048
  To Workspace : ToWorkspace  VariableName=alpha  SaveFormat=Timeseries  SampleTime=-1
  V : Outport
  alpha : Outport  Port=2
  beta : Outport  Port=3
  "Vb, rel" : Outport  Port=4
  wires:
  Sum/1 -> "Vb, rel"/1, "Incidence, Sideslip, & Airspeed"/1
  "Incidence, Sideslip, & Airspeed"/3 -> V/1
  "Incidence, Sideslip, & Airspeed"/1 -> alpha/1
  "Incidence, Sideslip, & Airspeed"/2 -> To Workspace/1, Scope1/1, beta/1
  h/1 -> Switch/2, Mux/3
  Mux/1 -> Horizontal Wind Model 14/1
  Constant1/1 -> Mux/2
  Constant/1 -> Mux/1
  Constant2/1 -> Horizontal Wind Model 14/2
  Constant3/1 -> Horizontal Wind Model 14/3
  Horizontal Wind Model 14/1 -> Switch/1
  Ground/1 -> Switch/3
  Switch/1 -> Mux1/2
  Ground1/1 -> Mux1/1
  Vb/1 -> Demux/1, Scope2/1, Sum/2
  Ground2/1 -> Horizontal Wind Model 14/4
  Mux1/1 -> Scope/1
  Discrete Wind Gust Model/1 -> Scope3/1
  Demux/1 -> Discrete Wind Gust Model/1
  Constant4/1 -> Mux2/2
  Re2b/1 -> Matrix Multiply/1
  Mux2/1 -> Matrix Multiply/2
  Matrix Multiply/1 -> Sum/3

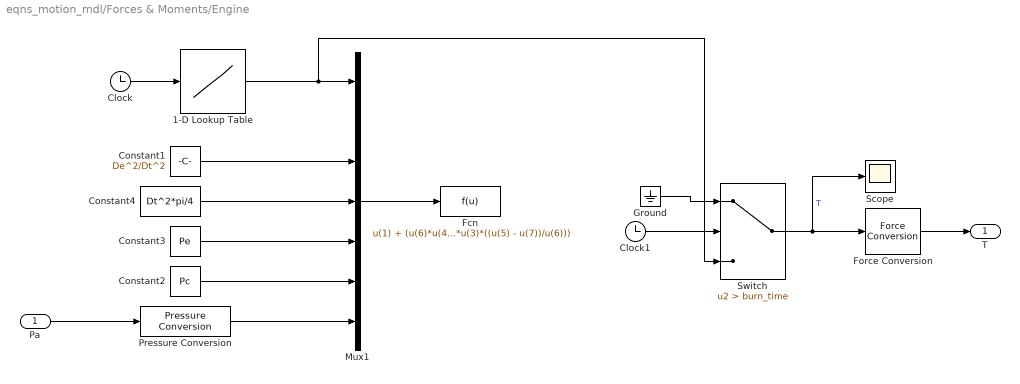
== system eqns_motion_mdl/Forces & Moments/Engine ==
  Pa : Inport
  1-D Lookup Table : Lookup_n-D  NumberOfTableDimensions=1  BreakpointsForDimension1=Thrust.time  Table=Thrust.thrust  InternalRulePriority=Speed  RndMeth=Simplest  InputSameDT=on
  Clock : Clock
  Clock1 : Clock
  Constant1 : Constant  Value=De^2/Dt^2
  Constant2 : Constant  Value=Pc
  Constant3 : Constant  Value=Pe
  Constant4 : Constant  Value=Dt^2*pi/4
  Fcn : Fcn  Expr=u(1) + (u(6)*u(4)*u(3)*((u(5) - u(7))/u(6)))
  Force Conversion : aerolibconvert2/Force Conversion  IU=lbf  OU=N
      settings: SourceProductName=Aerospace Blockset  SourceProductBaseCode=AE
  Ground : Ground
  Mux1 : Mux  Inputs=7
  Pressure Conversion : aerolibconvert2/Pressure Conversion  IU=Pa  OU=psi
      settings: SourceProductName=Aerospace Blockset  SourceProductBaseCode=AE
  Scope : Scope
  Switch : Switch  Criteria=u2 > Threshold  Threshold=burn_time
  T : Outport
  wires:
  Constant2/1 -> Mux1/6
  Constant3/1 -> Mux1/5
  Mux1/1 -> Fcn/1
  Constant1/1 -> Mux1/3
  Pa/1 -> Pressure Conversion/1
  Constant4/1 -> Mux1/4
  Switch/1 -> Force Conversion/1, Scope/1  "T"
  Force Conversion/1 -> T/1
  Pressure Conversion/1 -> Mux1/7
  Clock1/1 -> Switch/2
  Ground/1 -> Switch/1
  1-D Lookup Table/1 -> Switch/3, Mux1/1
  Clock/1 -> 1-D Lookup Table/1

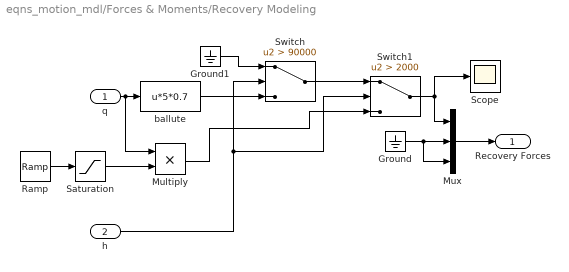
== system eqns_motion_mdl/Forces & Moments/Recovery Modeling ==
  q : Inport
  h : Inport  Port=2
  Ground : Ground
  Ground1 : Ground
  Multiply : Product
  Mux : Mux  Inputs=3
  Ramp : simulink/Sources/Ramp  slope=35.21  start=640  InitialOutput=0
  Saturation : Saturate  UpperLimit=65*0.65  LowerLimit=0
  Scope : Scope
  Switch : Switch  Criteria=u2 > Threshold  Threshold=90000
  Switch1 : Switch  Criteria=u2 > Threshold  Threshold=2000
  ballute : Fcn  Expr=u*5*0.7
  Recovery Forces : Outport
  wires:
  q/1 -> Multiply/1, ballute/1
  Mux/1 -> Recovery Forces/1
  Ground/1 -> Mux/3, Mux/2
  Ground1/1 -> Switch/1
  h/1 -> Switch1/2, Switch/2
  ballute/1 -> Switch/3
  Multiply/1 -> Switch1/3
  Switch/1 -> Switch1/1
  Switch1/1 -> Scope/1, Mux/1
  Ramp/1 -> Saturation/1
  Saturation/1 -> Multiply/2

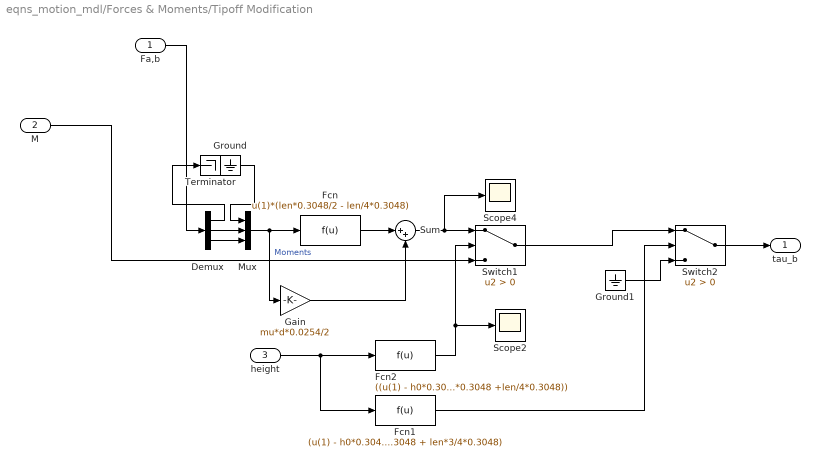
== system eqns_motion_mdl/Forces & Moments/Tipoff Modification ==
  Fa,b : Inport
  M : Inport  Port=2
  height : Inport  Port=3
  Demux : Demux  Outputs=3
  Fcn : Fcn  Expr=u(1)*(len*0.3048/2 - len/4*0.3048)
  Fcn1 : Fcn  Expr=(u(1) - h0*0.3048) > (lr*0.3048 + len*3/4*0.3048)
  Fcn2 : Fcn  Expr=((u(1) - h0*0.3048) > (lr*0.3048 + len*3/4*0.3048)) && ((u(1) - h0*0.3048) < (lr*0.3048 +len/4*0.3048))
  Gain : Gain  Gain=mu*d*0.0254/2
  Ground : Ground
  Ground1 : Ground
  Mux : Mux  Inputs=3
  Scope2 : Scope
  Scope4 : Scope
  Sum : Sum  Inputs=|++
  Switch1 : Switch  Criteria=u2 > Threshold
  Switch2 : Switch  Criteria=u2 > Threshold
  Terminator : Terminator
  tau_b : Outport
  wires:
  height/1 -> Fcn1/1, Fcn2/1
  Gain/1 -> Sum/2
  Switch1/1 -> Switch2/1
  Sum/1 -> Scope4/1, Switch1/1
  Fcn/1 -> Sum/1
  Fcn1/1 -> Switch2/2
  Ground/1 -> Mux/1
  M/1 -> Switch1/3  "Moments"
  Demux/1 -> Terminator/1
  Demux/3 -> Mux/3
  Mux/1 -> Gain/1, Fcn/1
  Switch2/1 -> tau_b/1
  Demux/2 -> Mux/2
  Ground1/1 -> Switch2/3
  Fa,b/1 -> Demux/1
  Fcn2/1 -> Switch1/2, Scope2/1

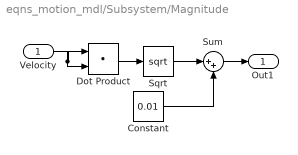
== system eqns_motion_mdl/Subsystem/Magnitude ==
  Velocity : Inport
  Constant : Constant  Value=0.01
  Dot Product : DotProduct  InputSameDT=on  OutDataTypeStr=Inherit: Inherit via internal rule
  Sqrt : Sqrt  SaturateOnIntegerOverflow=on
  Sum : Sum  Inputs=|++
  Out1 : Outport
  wires:
  Sum/1 -> Out1/1
  Velocity/1 -> Dot Product/2, Dot Product/1
  Dot Product/1 -> Sqrt/1
  Constant/1 -> Sum/2
  Sqrt/1 -> Sum/1
